simulink model "gtm_designFS"  (Simulink 8.0)
settings: Solver=ode3  SolverMode=SingleTasking  StartTime=0.0  StopTime=50  FixedStep=Timestep  MaxStep=0.1  MinStep=0.005  RelTol=1e-5
StopFcn:
  | MWSout=grabmws(bdroot);
  | MWSout.lastrun=datestr(now);
model workspace: external: MATLAB Code tmpfile_simWS.mat (data not in the file)
undefined symbols (not defined in the file): Aero, b, bias, INU_pos, LinearizeModeOn, runway_alt, sgn, sigbuilder_block, sldvsubsys, StatesInp, symmetric_aero_on, TrimModeOn
libraries: NoiseModel_lib x28, simulink x9, GTM_FS_aerolib x3, engine_GTM_FS_lib x2, Glenn_simp2_engine_lib x2, sensors_T2_lib x2, sldvlib x2, acparams_lib x1, auxvars_lib x1, eomlib x1, actuator_FS_lib x1, Coefficient_Evaluation_lib x1
(part 2 of 3)

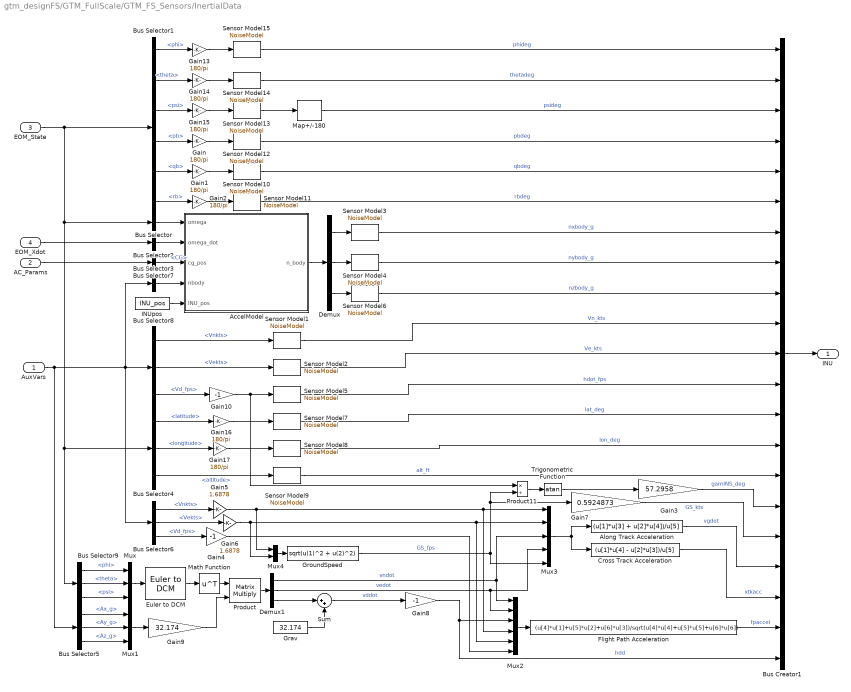
== system gtm_designFS/GTM_FullScale/GTM_FS_Sensors/InertialData ==
  AuxVars : Inport
  AC_Params : Inport  Port=2
  EOM_State : Inport  Port=3
  EOM_Xdot : Inport  Port=4
  AccelModel : MATLAB Function  TreatAsAtomicUnit=on
  Along Track Acceleration : Fcn  Expr=(u[1]*u[3] + u[2]*u[4])/u[5]
  Bus Creator1 : BusCreator  Inputs=21
  Bus Selector : BusSelector  OutputSignals=pb,qb,rb  OutputAsBus=on
  Bus Selector1 : BusSelector  OutputSignals=phi,theta,psi,pb,qb,rb
  Bus Selector2 : BusSelector  OutputSignals=pb_dot,qb_dot,rb_dot  OutputAsBus=on
  Bus Selector3 : BusSelector  OutputSignals=Ax_g,Ay_g,Az_g  OutputAsBus=on
  Bus Selector4 : BusSelector  OutputSignals=latitude,longitude,altitude
  Bus Selector5 : BusSelector  OutputSignals=Ax_g,Ay_g,Az_g
  Bus Selector6 : BusSelector  OutputSignals=Vnkts,Vekts,Vd_fps
  Bus Selector7 : BusSelector  OutputSignals=CG
  Bus Selector8 : BusSelector  OutputSignals=Vnkts,Vekts,Vd_fps
  Bus Selector9 : BusSelector  OutputSignals=phi,theta,psi
  Cross Track Acceleration : Fcn  Expr=(u[1]*u[4] - u[2]*u[3])/u[5]
  Demux : Demux  Outputs=3
  Demux1 : Demux  Outputs=3
  Euler to DCM : Euler_to_DCM_lib/Euler to DCM
  Flight Path Acceleration : Fcn  Expr=(u[4]*u[1]+u[5]*u[2]+u[6]*u[3])/sqrt(u[4]*u[4]+u[5]*u[5]+u[6]*u[6])
  Gain{,1..2,13..17} (8 alike) : Gain  Gain=180/pi
  Gain10 : Gain  Gain=-1
  Gain3 : Gain  Gain=57.2958  SaturateOnIntegerOverflow=on  OutDataTypeStr=Inherit: Same as input  ParamDataTypeStr=Inherit: Same as input
  Gain4 : Gain  Gain=-1
  Gain5 : Gain  Gain=1.6878
  Gain6 : Gain  Gain=1.6878
  Gain7 : Gain  Gain=0.5924873  SaturateOnIntegerOverflow=on  OutDataTypeStr=Inherit: Same as input  ParamDataTypeStr=Inherit: Same as input
  Gain8 : Gain  Gain=-1  SaturateOnIntegerOverflow=on  OutDataTypeStr=Inherit: Same as input  ParamDataTypeStr=Inherit: Same as input
  Gain9 : Gain  Gain=32.174  SaturateOnIntegerOverflow=on  OutDataTypeStr=Inherit: Same as input  ParamDataTypeStr=Inherit: Same as input
  Grav : Constant  Value=32.174  VectorParams1D=off
  GroundSpeed : Fcn  Expr=sqrt(u(1)^2 + u(2)^2)
  INUpos : Constant  Value=INU_pos  VectorParams1D=off
  Map+/-180 : sensors_T2_lib/GTM_T2/MIDG II 50 Hz/Map+//-180
  Math Function : Math  Operator=transpose  SaturateOnIntegerOverflow=on
  Mux : Mux  Inputs=3
  Mux1 : Mux  Inputs=3
  Mux2 : Mux  Inputs=6
  Mux3 : Mux  Inputs=5
  Mux4 : Mux  Inputs=2
  Product : Product  Multiplication=Matrix(*)  RndMeth=Zero
  Product11 : Product  Inputs=*/  SaturateOnIntegerOverflow=on  RndMeth=Zero  InputSameDT=on  OutDataTypeStr=Inherit: Same as first input
  Sensor Model1 : NoiseModel_lib/NoiseModel  noise_on=SensorNoise.On  sigma=SensorNoise.INU.Vn.Std  seed=878234  bias=SensorNoise.INU.Vn.Bias  scf=SensorNoise.INU.Vn.Scf
  Sensor Model10 : NoiseModel_lib/NoiseModel  noise_on=SensorNoise.On  sigma=SensorNoise.INU.qdeg.Std  seed=871234  bias=SensorNoise.INU.qdeg.Bias  scf=SensorNoise.INU.qdeg.Scf
  Sensor Model11 : NoiseModel_lib/NoiseModel  noise_on=SensorNoise.On  sigma=SensorNoise.INU.rdeg.Std  seed=878134  bias=SensorNoise.INU.rdeg.Bias  scf=SensorNoise.INU.rdeg.Scf
  Sensor Model12 : NoiseModel_lib/NoiseModel  noise_on=SensorNoise.On  sigma=SensorNoise.INU.pdeg.Std  seed=878233  bias=SensorNoise.INU.pdeg.Bias  scf=SensorNoise.INU.pdeg.Scf
  Sensor Model13 : NoiseModel_lib/NoiseModel  noise_on=SensorNoise.On  sigma=SensorNoise.INU.psi.Std  seed=878232  bias=SensorNoise.INU.psi.Bias  scf=SensorNoise.INU.psi.Scf
  Sensor Model14 : NoiseModel_lib/NoiseModel  noise_on=SensorNoise.On  sigma=SensorNoise.INU.theta.Std  seed=878231  bias=SensorNoise.INU.theta.Bias  scf=SensorNoise.INU.theta.Scf
  Sensor Model15 : NoiseModel_lib/NoiseModel  noise_on=SensorNoise.On  sigma=SensorNoise.INU.phi.Std  seed=878230  bias=SensorNoise.INU.phi.Bias  scf=SensorNoise.INU.phi.Scf
  Sensor Model2 : NoiseModel_lib/NoiseModel  noise_on=SensorNoise.On  sigma=SensorNoise.INU.Ve.Std  seed=8782345  bias=SensorNoise.INU.Ve.Bias  scf=SensorNoise.INU.Ve.Scf
  Sensor Model3 : NoiseModel_lib/NoiseModel  noise_on=SensorNoise.On  sigma=SensorNoise.INU.nxbody.Std  seed=878234  bias=SensorNoise.INU.nxbody.Bias  scf=SensorNoise.INU.nxbody.Scf
  Sensor Model4 : NoiseModel_lib/NoiseModel  noise_on=SensorNoise.On  sigma=SensorNoise.INU.nybody.Std  seed=8782345  bias=SensorNoise.INU.nybody.Bias  scf=SensorNoise.INU.nybody.Scf
  Sensor Model5 : NoiseModel_lib/NoiseModel  noise_on=SensorNoise.On  sigma=SensorNoise.INU.hdot.Std  seed=8782345  bias=SensorNoise.INU.hdot.Bias  scf=SensorNoise.INU.hdot.Scf
  Sensor Model6 : NoiseModel_lib/NoiseModel  noise_on=SensorNoise.On  sigma=SensorNoise.INU.nzbody.Std  seed=878236  bias=SensorNoise.INU.nzbody.Bias  scf=SensorNoise.INU.nzbody.Scf
  Sensor Model7 : NoiseModel_lib/NoiseModel  noise_on=SensorNoise.On  sigma=SensorNoise.INU.lat.Std  seed=8782345  bias=SensorNoise.INU.lat.Bias  scf=SensorNoise.INU.lat.Scf
  Sensor Model8 : NoiseModel_lib/NoiseModel  noise_on=SensorNoise.On  sigma=SensorNoise.INU.lon.Std  seed=8782345  bias=SensorNoise.INU.lon.Bias  scf=SensorNoise.INU.lon.Scf
  Sensor Model9 : NoiseModel_lib/NoiseModel  noise_on=SensorNoise.On  sigma=SensorNoise.INU.alt.Std  seed=8782345  bias=SensorNoise.INU.alt.Bias  scf=SensorNoise.INU.alt.Scf
  Sum : Sum  Inputs=|++
  Trigonometric Function : Trigonometry  Operator=atan
  INU : Outport
  wires:
  Bus Selector/1 -> AccelModel/1(omega)
  Bus Selector2/1 -> AccelModel/2(omega_dot)
  Bus Selector7/1 -> AccelModel/3(cg_pos)  "<CG>"
  Bus Selector3/1 -> AccelModel/4(nbody)
  AccelModel/1(n_body) -> Demux/1
  Demux/1 -> Sensor Model3/1
  Demux/2 -> Sensor Model4/1
  Demux/3 -> Sensor Model6/1
  Sensor Model1/1 -> Bus Creator1/10  "Vn_kts"
  Sensor Model2/1 -> Bus Creator1/11  "Ve_kts"
  Sensor Model9/1 -> Bus Creator1/15  "alt_ft"
  Sensor Model7/1 -> Bus Creator1/13  "lat_deg"
  Sensor Model8/1 -> Bus Creator1/14  "lon_deg"
  Bus Selector8/1 -> Sensor Model1/1  "<Vnkts>"
  Bus Selector8/2 -> Sensor Model2/1  "<Vekts>"
  Bus Selector8/3 -> Gain10/1  "<Vd_fps>"
  Bus Selector4/1 -> Gain16/1  "<latitude>"
  Bus Selector4/2 -> Gain17/1  "<longitude>"
  Bus Selector4/3 -> Sensor Model9/1  "<altitude>"
  Sensor Model5/1 -> Bus Creator1/12  "hdot_fps"
  Gain16/1 -> Sensor Model7/1
  Gain17/1 -> Sensor Model8/1
  EOM_Xdot/1 -> Bus Selector2/1
  AC_Params/1 -> Bus Selector7/1
  AuxVars/1 -> Bus Selector8/1, Bus Selector3/1, Bus Selector6/1, Bus Selector5/1
  EOM_State/1 -> Bus Selector1/1, Bus Selector/1, Bus Selector4/1, Bus Selector9/1
  Bus Selector1/1 -> Gain13/1  "<phi>"
  Bus Selector1/2 -> Gain14/1  "<theta>"
  Bus Selector1/3 -> Gain15/1  "<psi>"
  Bus Selector1/4 -> Gain/1  "<pb>"
  Bus Selector1/5 -> Gain1/1  "<qb>"
  Bus Selector1/6 -> Gain2/1  "<rb>"
  Gain2/1 -> Sensor Model11/1
  Gain1/1 -> Sensor Model10/1
  Gain/1 -> Sensor Model12/1
  Gain15/1 -> Sensor Model13/1
  Gain14/1 -> Sensor Model14/1
  Gain13/1 -> Sensor Model15/1
  Sensor Model13/1 -> Map+/-180/1
  Sensor Model15/1 -> Bus Creator1/1  "phideg"
  Sensor Model14/1 -> Bus Creator1/2  "thetadeg"
  Map+/-180/1 -> Bus Creator1/3  "psideg"
  Sensor Model12/1 -> Bus Creator1/4  "pbdeg"
  Sensor Model10/1 -> Bus Creator1/5  "qbdeg"
  Sensor Model11/1 -> Bus Creator1/6  "rbdeg"
  Sensor Model3/1 -> Bus Creator1/7  "nxbody_g"
  Sensor Model4/1 -> Bus Creator1/8  "nybody_g"
  Sensor Model6/1 -> Bus Creator1/9  "nzbody_g"
  INUpos/1 -> AccelModel/5(INU_pos)
  Mux/1 -> Euler to DCM/1
  Euler to DCM/1 -> Math Function/1
  Bus Selector5/1 -> Mux1/1  "<Ax_g>"
  Bus Selector5/2 -> Mux1/2  "<Ay_g>"
  Bus Selector5/3 -> Mux1/3  "<Az_g>"
  Math Function/1 -> Product/1
  Mux1/1 -> Gain9/1
  Mux3/1 -> Cross Track Acceleration/1, Along Track Acceleration/1
  Mux2/1 -> Flight Path Acceleration/1
  Trigonometric Function/1 -> Gain3/1
  Product11/1 -> Trigonometric Function/1
  Bus Selector6/3 -> Gain4/1  "<Vd_fps>"
  Bus Selector6/1 -> Gain5/1  "<Vnkts>"
  Bus Selector6/2 -> Gain6/1  "<Vekts>"
  Product/1 -> Demux1/1
  Bus Selector9/1 -> Mux/1  "<phi>"
  Bus Selector9/2 -> Mux/2  "<theta>"
  Bus Selector9/3 -> Mux/3  "<psi>"
  Gain5/1 -> Mux4/1, Mux3/1, Mux2/4
  Gain6/1 -> Mux4/2, Mux3/2, Mux2/5
  Mux4/1 -> GroundSpeed/1
  GroundSpeed/1 -> Mux3/5, Product11/2, Gain7/1  "GS_fps"
  Demux1/1 -> Mux3/3, Mux2/1  "vndot"
  Demux1/2 -> Mux3/4, Mux2/2  "vedot"
  Gain3/1 -> Bus Creator1/16  "gamINS_deg"
  Along Track Acceleration/1 -> Bus Creator1/18  "vgdot"
  Cross Track Acceleration/1 -> Bus Creator1/19  "xtkacc"
  Flight Path Acceleration/1 -> Bus Creator1/20  "fpaccel"
  Gain7/1 -> Bus Creator1/17  "GS_kts"
  Gain8/1 -> Mux2/3, Bus Creator1/21  "hdd"
  Gain4/1 -> Mux2/6
  Gain9/1 -> Product/2
  Demux1/3 -> Sum/1
  Grav/1 -> Sum/2
  Sum/1 -> Gain8/1  "vddot"
  Bus Creator1/1 -> INU/1
  Gain10/1 -> Sensor Model5/1, Product11/1

== system gtm_designFS/GTM_FullScale/GTM_FS_Sensors/SurfaceData ==
  SurfacePos : Inport
  Bus Creator : BusCreator  Inputs=22
  Bus Selector : BusSelector  OutputSignals=ELLOB,ELLIB,ELROB,ELRIB,AILL,AILR,RUDU,RUDL,FLAPLIB,FLAPLOB,FLAPRIB,FLAPROB  OutputAsBus=on
  Bus Selector1 : BusSelector  OutputSignals=ELLOB,ELLIB,ELROB,ELRIB,AILL,AILR,RUDU,RUDL,FLAPLIB,FLAPLOB,FLAPRIB,FLAPROB
  Bus Selector2 : BusSelector  OutputSignals=SPLLIB,SPLLOB,SPLRIB,SPLROB,STAB,GEAR,BRAKE,THROTL,THROTR,STEER
  Sensor Model5 : NoiseModel_lib/NoiseModel  noise_on=SensorNoise.On  sigma=SensorNoise.pots.Std  seed=878239  bias=SensorNoise.pots.Bias  scf=SensorNoise.pots.Scf
  Surface Labels : sensors_T2_lib/GTM_T2/Surface Pots/Surface Labels
  SurfPos : Outport
  wires:
  Bus Selector/1 -> Sensor Model5/1
  SurfacePos/1 -> Bus Selector/1, Bus Selector2/1
  Sensor Model5/1 -> Surface Labels/1
  Bus Selector1/1 -> Bus Creator/1  "<ELLOB>"
  Bus Selector1/2 -> Bus Creator/2  "<ELLIB>"
  Bus Selector1/3 -> Bus Creator/3  "<ELROB>"
  Bus Selector1/4 -> Bus Creator/4  "<ELRIB>"
  Bus Selector1/5 -> Bus Creator/5  "<AILL>"
  Bus Selector1/6 -> Bus Creator/6  "<AILR>"
  Bus Selector1/7 -> Bus Creator/7  "<RUDU>"
  Bus Selector1/8 -> Bus Creator/8  "<RUDL>"
  Bus Selector1/9 -> Bus Creator/9  "<FLAPLIB>"
  Bus Selector1/10 -> Bus Creator/10  "<FLAPLOB>"
  Bus Selector1/11 -> Bus Creator/11  "<FLAPRIB>"
  Bus Selector1/12 -> Bus Creator/12  "<FLAPROB>"
  Bus Selector2/1 -> Bus Creator/13  "<SPLLIB>"
  Bus Selector2/2 -> Bus Creator/14  "<SPLLOB>"
  Bus Selector2/3 -> Bus Creator/15  "<SPLRIB>"
  Bus Selector2/4 -> Bus Creator/16  "<SPLROB>"
  Bus Selector2/5 -> Bus Creator/17  "<STAB>"
  Bus Selector2/6 -> Bus Creator/18  "<GEAR>"
  Bus Selector2/7 -> Bus Creator/19  "<BRAKE>"
  Bus Selector2/8 -> Bus Creator/20  "<THROTL>"
  Bus Selector2/9 -> Bus Creator/21  "<THROTR>"
  Bus Selector2/10 -> Bus Creator/22  "<STEER>"
  Surface Labels/1 -> Bus Selector1/1
  Bus Creator/1 -> SurfPos/1

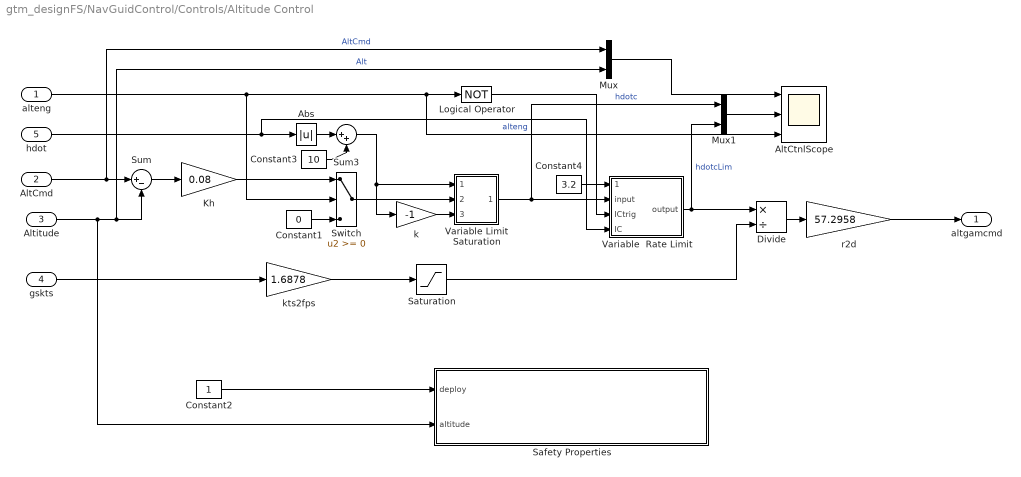
== system gtm_designFS/NavGuidControl/Controls/Altitude Control ==
  alteng : Inport
  AltCmd : Inport  Port=2
  Altitude : Inport  Port=3
  gskts : Inport  Port=4
  hdot : Inport  Port=5
  Abs : Abs  SaturateOnIntegerOverflow=on
  AltCtnlScope : Scope  NumInputPorts=3
      settings: TimeRange=30  YMin=10000~-5~0  YMax=10200~15~1  SaveName=ScopeData3
  Constant1 : Constant  Value=0
  Constant2 : Constant
  Constant3 : Constant  Value=10
  Constant4 : Constant  Value=3.2
  Divide : Product  Inputs=*/
  Kh : Gain  Gain=0.08
  Logical Operator : Logic  Operator=NOT
  Mux : Mux  Inputs=2
  Mux1 : Mux  Inputs=2
  Safety Properties : Subsystem  Tag=VerificationSubsystem  DisableCoverage=on  LoadFcn=sldvsubsys('check')  TreatAsAtomicUnit=on  SimViewingDevice=on  mask(VerificationSubsystem){}
      mask init:
      | sldvsubsys('maskInit');
      settings: CopyFcn=sldvsubsys('copy');  OpenFcn=open_system(gcb,'force');
      settings: PreSaveFcn=|
      | set_param(gcb,'SimViewingDevice','on');
      | sldvsubsys('check');
      mask Help: helpview(fullfile(docroot,'toolbox','sldv','sldv.map'),'verificationsubsystem')
      mask Display: image(imread('sldvicon_versubsys.png','BackGroundColor',[1 1 1]),'center');
  Saturation : Saturate  UpperLimit=1000  LowerLimit=0.0001
  Sum : Sum  Inputs=|+-
  Sum3 : Sum  Inputs=|++  SaturateOnIntegerOverflow=on  InputSameDT=on  OutDataTypeStr=Inherit: Same as first input
  Switch : Switch
  Variable  Rate Limit : Subsystem
  Variable Limit Saturation : Subsystem
  k : Gain  Gain=-1
  kts2fps : Gain  Gain=1.6878
  r2d : Gain  Gain=57.2958
  altgamcmd : Outport
  wires:
  Sum/1 -> Kh/1
  AltCmd/1 -> Sum/1, Mux/1  "AltCmd"
  Altitude/1 -> Safety Properties/2(altitude), Sum/2, Mux/2  "Alt"
  hdot/1 -> Abs/1, Variable  Rate Limit/4(IC)
  Abs/1 -> Sum3/1
  Constant3/1 -> Sum3/2
  k/1 -> Variable Limit Saturation/3(Lo_lim)
  Sum3/1 -> k/1, Variable Limit Saturation/1(up_lim)
  alteng/1 -> Switch/2, Logical Operator/1, AltCtnlScope/3  "alteng"
  gskts/1 -> kts2fps/1
  Divide/1 -> r2d/1
  r2d/1 -> altgamcmd/1
  Logical Operator/1 -> Variable  Rate Limit/3(ICtrig)
  Variable Limit Saturation/1(Out1) -> Variable  Rate Limit/2(input), Mux1/1  "hdotc"
  Constant4/1 -> Variable  Rate Limit/1(ratelim)
  Variable  Rate Limit/1(output) -> Divide/1, Mux1/2  "hdotcLim"
  kts2fps/1 -> Saturation/1
  Saturation/1 -> Divide/2
  Switch/1 -> Variable Limit Saturation/2(SigIn)
  Kh/1 -> Switch/1
  Constant1/1 -> Switch/3
  Mux/1 -> AltCtnlScope/1
  Mux1/1 -> AltCtnlScope/2
  Constant2/1 -> Safety Properties/1(deploy)

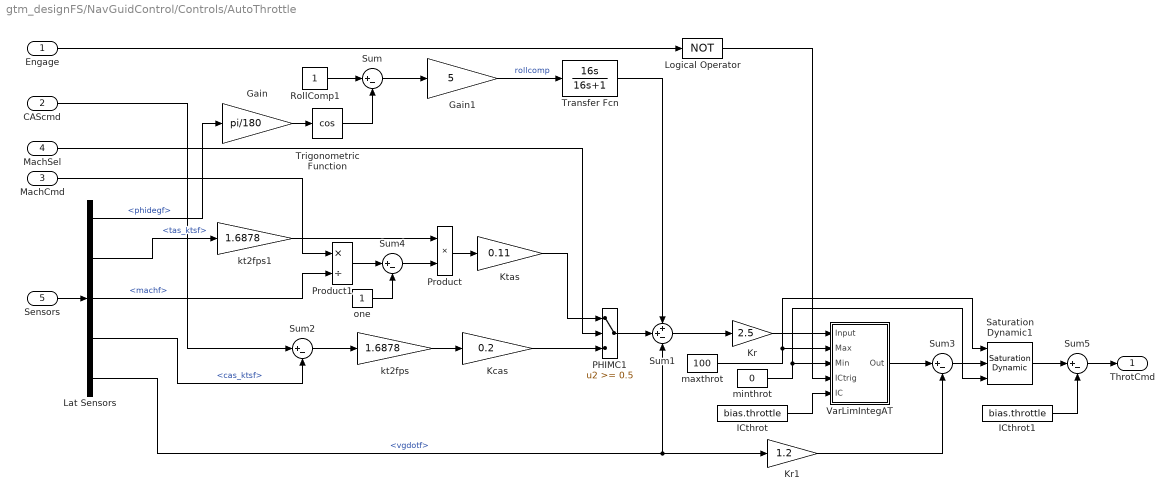
== system gtm_designFS/NavGuidControl/Controls/AutoThrottle ==
  Engage : Inport
  CAScmd : Inport  Port=2
  MachCmd : Inport  Port=3
  MachSel : Inport  Port=4
  Sensors : Inport  Port=5
  Gain : Gain  Gain=pi/180
  Gain1 : Gain  Gain=5
  ICthrot : Constant  Value=bias.throttle  SampleTime=-1
  ICthrot1 : Constant  Value=bias.throttle  SampleTime=-1
  Kcas : Gain  Gain=0.2
  Kr : Gain  Gain=2.5
  Kr1 : Gain  Gain=1.2
  Ktas : Gain  Gain=0.11
  Lat Sensors : BusSelector  OutputSignals=phidegf,tas_ktsf,machf,cas_ktsf,vgdotf
  Logical Operator : Logic  Operator=NOT  AllPortsSameDT=off  OutDataTypeStr=boolean
  PHIMC1 : Switch  Threshold=0.5  SampleTime=0.02  SaturateOnIntegerOverflow=on
  Product : Product  RndMeth=Zero
  Product1 : Product  Inputs=*/  RndMeth=Zero
  RollComp1 : Constant  SampleTime=-1
  Saturation Dynamic1 : simulink/Discontinuities/Saturation Dynamic  OutMin=[]  OutMax=[]  OutDataTypeStr=Inherit: Same as second input  OutDataType=sfix(16)  OutScaling=2^-10  DoSatur=off
  Sum{,2..5} (5 alike) : Sum  Inputs=|+-
  Sum1 : Sum  Inputs=++-
  Transfer Fcn : TransferFcn  Numerator=[16 0]  Denominator=[16 1]
  Trigonometric Function : Trigonometry  Operator=cos
  VarLimIntegAT : Subsystem
  kt2fps : Gain  Gain=1.6878
  kt2fps1 : Gain  Gain=1.6878
  maxthrot : Constant  Value=100  SampleTime=-1
  minthrot : Constant  Value=0  SampleTime=-1
  one : Constant  SampleTime=-1
  ThrotCmd : Outport
  wires:
  CAScmd/1 -> Sum2/1
  Sum2/1 -> kt2fps/1
  Sum1/1 -> Kr/1
  kt2fps/1 -> Kcas/1
  Kr/1 -> VarLimIntegAT/1(Input)
  Lat Sensors/5 -> Sum1/3, Kr1/1  "<vgdotf>"
  Kr1/1 -> Sum3/2
  Gain1/1 -> Transfer Fcn/1  "rollcomp"
  Sum/1 -> Gain1/1
  Trigonometric Function/1 -> Sum/2
  RollComp1/1 -> Sum/1
  Gain/1 -> Trigonometric Function/1
  Product1/1 -> Sum4/1
  one/1 -> Sum4/2
  Sum4/1 -> Product/2
  kt2fps1/1 -> Product/1
  Product/1 -> Ktas/1
  ICthrot/1 -> VarLimIntegAT/5(IC)
  Sum5/1 -> ThrotCmd/1
  ICthrot1/1 -> Sum5/2
  maxthrot/1 -> VarLimIntegAT/2(Max), Saturation Dynamic1/1
  minthrot/1 -> VarLimIntegAT/3(Min), Saturation Dynamic1/3
  VarLimIntegAT/1(Out) -> Sum3/1
  Sum3/1 -> Saturation Dynamic1/2
  Saturation Dynamic1/1 -> Sum5/1
  PHIMC1/1 -> Sum1/2
  Kcas/1 -> PHIMC1/3
  Ktas/1 -> PHIMC1/1
  Transfer Fcn/1 -> Sum1/1
  Sensors/1 -> Lat Sensors/1
  Lat Sensors/1 -> Gain/1  "<phidegf>"
  Lat Sensors/2 -> kt2fps1/1  "<tas_ktsf>"
  Lat Sensors/4 -> Sum2/2  "<cas_ktsf>"
  Logical Operator/1 -> VarLimIntegAT/4(ICtrig)
  Engage/1 -> Logical Operator/1
  MachSel/1 -> PHIMC1/2
  MachCmd/1 -> Product1/1
  Lat Sensors/3 -> Product1/2  "<machf>"

== system gtm_designFS/NavGuidControl/Controls/FPA Control ==
  engage : Inport
  gamcmd : Inport  Port=2
  gamma : Inport  Port=3
  thetadeg : Inport  Port=4
  VT : Inport  Port=5
  FPAScope : Scope  NumInputPorts=4
      settings: YMin=-1~-5~-2~-5  YMax=2~5~2~10  SaveName=ScopeData12
  Integ_FPA : Integrator  ExternalReset=level  InitialConditionSource=external  IgnoreLimit=on
  KIgamerr : Gain
  Kgamerr : Gain  Gain=1.4
  Logical Operator : Logic  Operator=NOT  AllPortsSameDT=off  OutDataTypeStr=boolean
  Mux : Mux  Inputs=2
  Mux1 : Mux  Inputs=2
  Product1 : Product  RndMeth=Zero
  Saturation Dynamic : simulink/Discontinuities/Saturation Dynamic  OutMin=[]  OutMax=[]  OutDataTypeStr=Inherit: Same as second input  OutDataType=fixdt(1, 16)  OutScaling=2^-10  DoSatur=off
  Sum : Sum  Inputs=|++
  Sum1 : Sum  Inputs=|+-
  Sum2 : Sum  Inputs=|+-
  hddLim : Constant  Value=4.83*57.2958
  kt2fps : Gain  Gain=1.6878
  m1 : Gain  Gain=-1
  PitchCmd : Outport
  wires:
  Sum1/1 -> PitchCmd/1, FPAScope/4  "PitchCmd"
  Kgamerr/1 -> Sum1/2, Sum/2
  Integ_FPA/1 -> Sum1/1
  gamma/1 -> Kgamerr/1, Sum2/2, Mux/2  "gamma"
  thetadeg/1 -> Sum/1
  Sum/1 -> Integ_FPA/3
  engage/1 -> Logical Operator/1, FPAScope/1  "engage"
  Logical Operator/1 -> Integ_FPA/2
  kt2fps/1 -> Product1/2
  hddLim/1 -> Product1/1
  Product1/1 -> Saturation Dynamic/1, m1/1
  VT/1 -> kt2fps/1
  Saturation Dynamic/1 -> Integ_FPA/1, Mux1/2  "gamerrlim"
  KIgamerr/1 -> Saturation Dynamic/2
  m1/1 -> Saturation Dynamic/3
  Sum2/1 -> KIgamerr/1, Mux1/1  "gamerr"
  gamcmd/1 -> Sum2/1, Mux/1  "gamcmd"
  Mux/1 -> FPAScope/2
  Mux1/1 -> FPAScope/3

== system gtm_designFS/NavGuidControl/Controls/FPAcmd ==
  Demux : Demux  Tag=STV Demux  Outputs=1
  FromWs : FromWorkspace  Tag=STV FromWs  VariableName=tuvar  SampleTime=0  SigBuilderData=DataTag0  VnvData=DataTag1
      SigBuilderData=|
      | common.afterFinalStr = 'Extrapolate'
      | common.sampleTime = 0
      | dataSet.timeRange = [0 10]
      | dataSet.name = 'Group 1'
      | sbobj.Groups.Name = 'Group 1'
      | sbobj.Groups.Signals.Name = 'Signal 1'
      | sbobj.Groups.Signals.XData = [0 1 1 6 10]
      | sbobj.Groups.Signals.YData = [0 0 1 1 1]
  Signal 1 : Outport  Tag=STV Outport
  wires:
  Demux/1 -> Signal 1/1
  FromWs/1 -> Demux/1

== system gtm_designFS/NavGuidControl/Controls/Heading Control ==
  HdgCmdMCP : Inport
  Heading : Inport  Port=2
  psidot : Inport  Port=3
  Vt : Inport  Port=4
  Roll : Inport  Port=5
  HdgCmdProcessor : Subsystem
  HdgRollCmdScope : Scope  NumInputPorts=8
      settings: YMin=-30~-30~-10~-10~-4~-10~0~-5  YMax=30~30~10~10~4~10~1~5  SaveName=ScopeData7
  Khdg : Gain  Gain=0.05
  Khdg1 : Gain
  Khdg2 : Gain
  Khdgrte : Gain  Gain=3
  Logical Operator : Logic  Operator=NOT  AllPortsSameDT=off  OutDataTypeStr=boolean
  MinMax : MinMax  Inputs=2
  MinMax1 : MinMax  Function=max  Inputs=2
  Mux : Mux  Inputs=2
  Sum : Sum  Inputs=|+-
  Sum1 : Sum  Inputs=|++
  Sum2 : Sum  Inputs=|+-
  Sum3 : Sum  Inputs=|--
  Sum4 : Sum  Inputs=+-|
  VarLimIntegIC : Subsystem
  sgn : Gain  Gain=-1
  RollCmd : Outport
  wires:
  Heading/1 -> Sum/2, HdgCmdProcessor/3(Heading)
  HdgCmdProcessor/1(HdgCmd) -> Sum/1, Mux/2  "psic"
  Sum/1 -> Khdg/1, HdgRollCmdScope/3  "psie"
  Khdg/1 -> Sum1/1
  Sum2/1 -> Sum1/2, HdgRollCmdScope/4  "psidote"
  HdgCmdProcessor/2(HdgRteCmd) -> Sum2/1, HdgRollCmdScope/2  "psidotc"
  psidot/1 -> Sum2/2
  Vt/1 -> HdgCmdProcessor/1(Vt)
  HdgCmdMCP/1 -> HdgCmdProcessor/2(HdgCmdMCP), Mux/1
  VarLimIntegIC/1(Out) -> RollCmd/1, Sum3/1, Sum4/2, HdgRollCmdScope/8  "phic"
  [rollLim] -> VarLimIntegIC/1(UpLim), sgn/1
  sgn/1 -> VarLimIntegIC/2(LoLim)
  [rollLim] -> Sum3/2, Sum4/1
  Sum1/1 -> Khdgrte/1
  MinMax1/1 -> MinMax/1, HdgRollCmdScope/6  "phidotcmx"
  MinMax/1 -> VarLimIntegIC/3(In), HdgRollCmdScope/7  "phidotcmn"
  [apeng] -> Logical Operator/1
  Sum3/1 -> Khdg1/1
  Sum4/1 -> Khdg2/1
  Khdg1/1 -> MinMax1/2
  Khdg2/1 -> MinMax/2
  Roll/1 -> VarLimIntegIC/5(IC)
  Khdgrte/1 -> MinMax1/1, HdgRollCmdScope/5  "phidotc"
  Logical Operator/1 -> VarLimIntegIC/4(Trig)
  Mux/1 -> HdgRollCmdScope/1

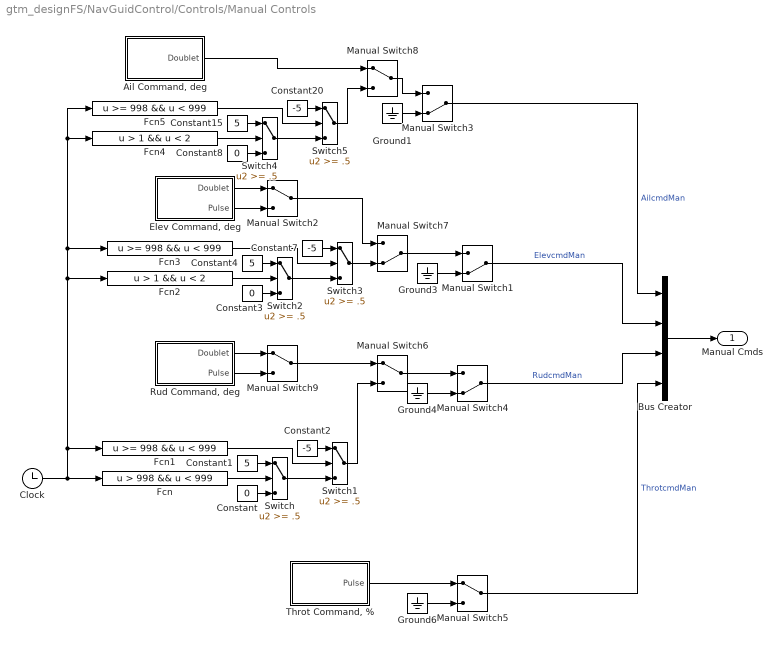
== system gtm_designFS/NavGuidControl/Controls/Manual Controls ==
  "Ail Command, deg" : Subsystem  Tag=STV Subsys  LoadFcn=sigbuilder_block('load');  StartFcn=sigbuilder_block('start');  StopFcn=sigbuilder_block('stop');  ClipboardFcn=sigbuilder_block('clipboard');  mask(Sigbuilder block){}
      mask help: Sigbuilder GUI
      mask init:
      | if ~strcmp(get_param(bdroot(gcbh),'SimulationStatus'),'stopped') tuvar = sigbuilder_block('maskInit'); end
      settings: CopyFcn=sigbuilder_block('copy');  DeleteFcn=sigbuilder_block('delete');  ModelCloseFcn=sigbuilder_block('modelClose');  PreSaveFcn=sigbuilder_block('preSave');  PauseFcn=sigbuilder_block('pause')  ContinueFcn=sigbuilder_block('continue')  NameChangeFcn=sigbuilder_block('namechange');  OpenFcn=sigbuilder_block('open',[20.16 261.12 550.08 400.32 ]);  CloseFcn=sigbuilder_block('close');
      mask Display: plot(0,0,100,100,[10,10,40,40,10],[80,20,20,80,80],[40,10],[50,50], [40,27,10],[65,72,56],[40,25,25,10],[28,28,43,43]);
  Bus Creator : BusCreator
  Clock : Clock
  Constant : Constant  Value=0
  Constant1 : Constant  Value=5
  Constant15 : Constant  Value=5
  Constant2 : Constant  Value=-5
  Constant20 : Constant  Value=-5
  Constant3 : Constant  Value=0
  Constant4 : Constant  Value=5
  Constant7 : Constant  Value=-5
  Constant8 : Constant  Value=0
  "Elev Command, deg" : Subsystem  Tag=STV Subsys  LoadFcn=sigbuilder_block('load');  StartFcn=sigbuilder_block('start');  StopFcn=sigbuilder_block('stop');  ClipboardFcn=sigbuilder_block('clipboard');  mask(Sigbuilder block){}
      mask help: Sigbuilder GUI
      mask init:
      | if ~strcmp(get_param(bdroot(gcbh),'SimulationStatus'),'stopped') tuvar = sigbuilder_block('maskInit'); end
      settings: CopyFcn=sigbuilder_block('copy');  DeleteFcn=sigbuilder_block('delete');  ModelCloseFcn=sigbuilder_block('modelClose');  PreSaveFcn=sigbuilder_block('preSave');  PauseFcn=sigbuilder_block('pause')  ContinueFcn=sigbuilder_block('continue')  NameChangeFcn=sigbuilder_block('namechange');  OpenFcn=sigbuilder_block('open',[550.08 198.72 550.08 400.32 ]);  CloseFcn=sigbuilder_block('close');
      mask Display: plot(0,0,100,100,[10,10,40,40,10],[80,20,20,80,80],[40,10],[50,50], [40,27,10],[65,72,56],[40,25,25,10],[28,28,43,43]);
  Fcn : Fcn  Expr=u > 998 && u < 999
  Fcn1 : Fcn  Expr=u >= 998 && u < 999
  Fcn2 : Fcn  Expr=u > 1 && u < 2
  Fcn3 : Fcn  Expr=u >= 998 && u < 999
  Fcn4 : Fcn  Expr=u > 1 && u < 2
  Fcn5 : Fcn  Expr=u >= 998 && u < 999
  Ground{1,3..4,6} (4 alike) : Ground
  Manual Switch{1,3..4,7} (4 alike) : ManualSwitch  CurrentSetting=0
  Manual Switch{2,5..6,8..9} (5 alike) : ManualSwitch
  "Rud Command, deg" : Subsystem  Tag=STV Subsys  LoadFcn=sigbuilder_block('load');  StartFcn=sigbuilder_block('start');  StopFcn=sigbuilder_block('stop');  ClipboardFcn=sigbuilder_block('clipboard');  mask(Sigbuilder block){}
      mask help: Sigbuilder GUI
      mask init:
      | if ~strcmp(get_param(bdroot(gcbh),'SimulationStatus'),'stopped') tuvar = sigbuilder_block('maskInit'); end
      settings: CopyFcn=sigbuilder_block('copy');  DeleteFcn=sigbuilder_block('delete');  ModelCloseFcn=sigbuilder_block('modelClose');  PreSaveFcn=sigbuilder_block('preSave');  PauseFcn=sigbuilder_block('pause')  ContinueFcn=sigbuilder_block('continue')  NameChangeFcn=sigbuilder_block('namechange');  OpenFcn=sigbuilder_block('open',[437.6 199.2 550.4 400 ]);  CloseFcn=sigbuilder_block('close');
      mask Display: plot(0,0,100,100,[10,10,40,40,10],[80,20,20,80,80],[40,10],[50,50], [40,27,10],[65,72,56],[40,25,25,10],[28,28,43,43]);
  Switch{,1..5} (6 alike) : Switch  Threshold=.5
  "Throt Command, %" : Subsystem  Tag=STV Subsys  LoadFcn=sigbuilder_block('load');  StartFcn=sigbuilder_block('start');  StopFcn=sigbuilder_block('stop');  ClipboardFcn=sigbuilder_block('clipboard');  mask(Sigbuilder block){}
      mask help: Sigbuilder GUI
      mask init:
      | if ~strcmp(get_param(bdroot(gcbh),'SimulationStatus'),'stopped') tuvar = sigbuilder_block('maskInit'); end
      settings: CopyFcn=sigbuilder_block('copy');  DeleteFcn=sigbuilder_block('delete');  ModelCloseFcn=sigbuilder_block('modelClose');  PreSaveFcn=sigbuilder_block('preSave');  PauseFcn=sigbuilder_block('pause')  ContinueFcn=sigbuilder_block('continue')  NameChangeFcn=sigbuilder_block('namechange');  OpenFcn=sigbuilder_block('open',[436.656 201.841 549.567 399.685 ]);  CloseFcn=sigbuilder_block('close');
      mask Display: plot(0,0,100,100,[10,10,40,40,10],[80,20,20,80,80],[40,10],[50,50], [40,27,10],[65,72,56],[40,25,25,10],[28,28,43,43]);
  Manual Cmds : Outport
  wires:
  Ground1/1 -> Manual Switch3/2
  Ground3/1 -> Manual Switch1/2
  "Elev Command, deg"/1(Doublet) -> Manual Switch2/1
  "Elev Command, deg"/2(Pulse) -> Manual Switch2/2
  Ground4/1 -> Manual Switch4/2
  Ground6/1 -> Manual Switch5/2
  "Throt Command, %"/1(Pulse) -> Manual Switch5/1
  Fcn/1 -> Switch/2
  Constant1/1 -> Switch/1
  Constant/1 -> Switch/3
  Switch/1 -> Switch1/3
  Constant2/1 -> Switch1/1
  Fcn1/1 -> Switch1/2
  Clock/1 -> Fcn/1, Fcn1/1, Fcn2/1, Fcn3/1, Fcn5/1, Fcn4/1
  Manual Switch6/1 -> Manual Switch4/1
  Switch1/1 -> Manual Switch6/2
  Fcn2/1 -> Switch2/2
  Constant4/1 -> Switch2/1
  Constant3/1 -> Switch2/3
  Switch2/1 -> Switch3/3
  Constant7/1 -> Switch3/1
  Fcn3/1 -> Switch3/2
  Manual Switch7/1 -> Manual Switch1/1
  Switch3/1 -> Manual Switch7/2
  Manual Switch2/1 -> Manual Switch7/1
  Fcn4/1 -> Switch4/2
  Constant15/1 -> Switch4/1
  Constant8/1 -> Switch4/3
  Switch4/1 -> Switch5/3
  Constant20/1 -> Switch5/1
  Fcn5/1 -> Switch5/2
  Manual Switch8/1 -> Manual Switch3/1
  Switch5/1 -> Manual Switch8/2
  "Ail Command, deg"/1(Doublet) -> Manual Switch8/1
  Manual Switch3/1 -> Bus Creator/1  "AilcmdMan"
  Manual Switch1/1 -> Bus Creator/2  "ElevcmdMan"
  Manual Switch4/1 -> Bus Creator/3  "RudcmdMan"
  Manual Switch5/1 -> Bus Creator/4  "ThrotcmdMan"
  Bus Creator/1 -> Manual Cmds/1
  "Rud Command, deg"/1(Doublet) -> Manual Switch9/1
  "Rud Command, deg"/2(Pulse) -> Manual Switch9/2
  Manual Switch9/1 -> Manual Switch6/1

== system gtm_designFS/NavGuidControl/Controls/ManualPitchcmd ==
  Thetafiltdeg : Inport
  Constant : Constant  Value=3
  Constant1 : Constant  Value=0
  Integrator +/- 50 deg/sec : Integrator  InitialConditionSource=external  LimitOutput=on  UpperSaturationLimit=50  LowerSaturationLimit=-50
  ManualPitchScope : Scope  NumInputPorts=6
      settings: YMin=-5~-5~-5~-5~-5~-5  YMax=5~5~5~5~5~5  SaveName=ScopeData8
  Multiport Switch : MultiPortSwitch
  PS Gain deg/sec : Gain  Gain=50
  "PS Shaping " : Fcn  Expr=u(1)*abs(u(1))^1.0
  PS deadband +/- 0.01 : DeadZone  LowerValue=-0.01  UpperValue=0.01  SaturateOnIntegerOverflow=on
  PS limits +/- 1 : Saturate  UpperLimit=1  LowerLimit=-1
  Pitchcmd : Subsystem  Tag=STV Subsys  LoadFcn=sigbuilder_block('load');  StartFcn=sigbuilder_block('start');  StopFcn=sigbuilder_block('stop');  ClipboardFcn=sigbuilder_block('clipboard');  mask(Sigbuilder block){}
      mask help: Sigbuilder GUI
      mask init:
      | if ~strcmp(get_param(bdroot(gcbh),'SimulationStatus'),'stopped') tuvar = sigbuilder_block('maskInit'); end
      settings: CopyFcn=sigbuilder_block('copy');  DeleteFcn=sigbuilder_block('delete');  ModelCloseFcn=sigbuilder_block('modelClose');  PreSaveFcn=sigbuilder_block('preSave');  PauseFcn=sigbuilder_block('pause')  ContinueFcn=sigbuilder_block('continue')  NameChangeFcn=sigbuilder_block('namechange');  OpenFcn=sigbuilder_block('open',[159.36 418.56 676.8 484.8 ]);  CloseFcn=sigbuilder_block('close');
      mask Display: plot(0,0,100,100,[10,10,40,40,10],[80,20,20,80,80],[40,10],[50,50], [40,27,10],[65,72,56],[40,25,25,10],[28,28,43,43]);
  PitchCmd : Outport
  wires:
  Pitchcmd/2(Signal 2) -> Multiport Switch/4
  Pitchcmd/1(Signal 1) -> Multiport Switch/3
  Constant1/1 -> Multiport Switch/2
  Constant/1 -> Multiport Switch/1
  Multiport Switch/1 -> ManualPitchScope/1, PS limits +/- 1/1  "stick"
  Thetafiltdeg/1 -> Integrator +/- 50 deg/sec/2
  Integrator +/- 50 deg/sec/1 -> ManualPitchScope/6, PitchCmd/1  "pitchcmd"
  PS Gain deg/sec/1 -> ManualPitchScope/5, Integrator +/- 50 deg/sec/1  "q_cmd"
  PS deadband +/- 0.01/1 -> ManualPitchScope/3, "PS Shaping "/1  "stkdb"
  PS limits +/- 1/1 -> ManualPitchScope/2, PS deadband +/- 0.01/1  "stklim"
  "PS Shaping "/1 -> ManualPitchScope/4, PS Gain deg/sec/1  "stkshape"

== system gtm_designFS/NavGuidControl/Controls/ManualRollcmd ==
  rollfiltdeg : Inport
  Constant1 : Constant  Value=0
  Integrator +/- 225 deg/sec : Integrator  InitialConditionSource=external  LimitOutput=on  UpperSaturationLimit=225  LowerSaturationLimit=-225
  ManualRollScope : Scope  NumInputPorts=6
      settings: YMin=-5~-5~-5~-5~-5~-5  YMax=5~5~5~5~5~5  SaveName=ScopeData9
  Multiport Switch : MultiPortSwitch
  RS Gain deg/sec : Gain  Gain=225
  "RS Shaping " : Fcn  Expr=u(1)*abs(u(1))^1.0
  RS deadband +/- 0.01 : DeadZone  LowerValue=-0.01  UpperValue=0.01  SaturateOnIntegerOverflow=on
  RS limits +/- 1 : Saturate  UpperLimit=1  LowerLimit=-1
  Rollcmd : Subsystem  Tag=STV Subsys  LoadFcn=sigbuilder_block('load');  StartFcn=sigbuilder_block('start');  StopFcn=sigbuilder_block('stop');  ClipboardFcn=sigbuilder_block('clipboard');  mask(Sigbuilder block){}
      mask help: Sigbuilder GUI
      mask init:
      | if ~strcmp(get_param(bdroot(gcbh),'SimulationStatus'),'stopped') tuvar = sigbuilder_block('maskInit'); end
      settings: CopyFcn=sigbuilder_block('copy');  DeleteFcn=sigbuilder_block('delete');  ModelCloseFcn=sigbuilder_block('modelClose');  PreSaveFcn=sigbuilder_block('preSave');  PauseFcn=sigbuilder_block('pause')  ContinueFcn=sigbuilder_block('continue')  NameChangeFcn=sigbuilder_block('namechange');  OpenFcn=sigbuilder_block('open',[159.36 418.56 676.8 484.8 ]);  CloseFcn=sigbuilder_block('close');
      mask Display: plot(0,0,100,100,[10,10,40,40,10],[80,20,20,80,80],[40,10],[50,50], [40,27,10],[65,72,56],[40,25,25,10],[28,28,43,43]);
  portselect : Constant
  RollCmd : Outport
  wires:
  rollfiltdeg/1 -> Integrator +/- 225 deg/sec/2
  Rollcmd/2(Signal 2) -> Multiport Switch/4
  Rollcmd/1(Signal 1) -> Multiport Switch/3
  Constant1/1 -> Multiport Switch/2
  Multiport Switch/1 -> ManualRollScope/1, RS limits +/- 1/1  "rollstick"
  Integrator +/- 225 deg/sec/1 -> ManualRollScope/6, RollCmd/1  "rollcmd"
  RS Gain deg/sec/1 -> ManualRollScope/5, Integrator +/- 225 deg/sec/1  "p_cmd"
  RS deadband +/- 0.01/1 -> ManualRollScope/3, "RS Shaping "/1  "rstkdb"
  RS limits +/- 1/1 -> ManualRollScope/2, RS deadband +/- 0.01/1  "rstklim"
  "RS Shaping "/1 -> ManualRollScope/4, RS Gain deg/sec/1  "rstkshape"
  portselect/1 -> Multiport Switch/1

== system gtm_designFS/NavGuidControl/Controls/Pitch InnerLoop ==
  PitchCmd : Inport
  Pitch : Inport  Port=2
  qdeg : Inport  Port=3
  CAS : Inport  Port=4
  Kcas : Lookup  InputValues=[0 120 350 500]  Table=[1.0 1.0 0.3 0.3]
  Kpitch : Gain  Gain=2
  Kwo : Gain  Gain=0.5
  Mux : Mux  Inputs=2
  PitchScope : Scope  NumInputPorts=6
      settings: YMin=-2~-2~-2~-20~-20~0  YMax=10~2~2~20~20~1.2  SaveName=ScopeData11
  Product : Product  RndMeth=Zero
  Sum : Sum  Inputs=|+-
  Sum1 : Sum  Inputs=|-+
  Transfer Fcn : TransferFcn  Numerator=[16 0]  Denominator=[16 1]
  ElevCmd : Outport
  wires:
  Sum/1 -> Kpitch/1, PitchScope/2  "Pitcherror"
  Pitch/1 -> Sum/2, Mux/2
  Kpitch/1 -> Sum1/1
  qdeg/1 -> Transfer Fcn/1
  Transfer Fcn/1 -> Kwo/1
  CAS/1 -> Kcas/1
  Sum1/1 -> Product/1, PitchScope/4  "dec"
  Kcas/1 -> Product/2, PitchScope/6  "Kcas"
  Product/1 -> ElevCmd/1, PitchScope/5  "elevcmd"
  Kwo/1 -> Sum1/2, PitchScope/3  "qdegwo"
  PitchCmd/1 -> Sum/1, Mux/1  "Pitchcmd"
  Mux/1 -> PitchScope/1

== system gtm_designFS/NavGuidControl/Controls/PitchCmd ==
  Pitchcmd1 : Subsystem  Tag=STV Subsys  LoadFcn=sigbuilder_block('load');  StartFcn=sigbuilder_block('start');  StopFcn=sigbuilder_block('stop');  ClipboardFcn=sigbuilder_block('clipboard');  mask(Sigbuilder block){}
      mask help: Sigbuilder GUI
      mask init:
      | if ~strcmp(get_param(bdroot(gcbh),'SimulationStatus'),'stopped') tuvar = sigbuilder_block('maskInit'); end
      settings: CopyFcn=sigbuilder_block('copy');  DeleteFcn=sigbuilder_block('delete');  ModelCloseFcn=sigbuilder_block('modelClose');  PreSaveFcn=sigbuilder_block('preSave');  PauseFcn=sigbuilder_block('pause')  ContinueFcn=sigbuilder_block('continue')  NameChangeFcn=sigbuilder_block('namechange');  OpenFcn=sigbuilder_block('open',[437.6 199.2 550.4 400 ]);  CloseFcn=sigbuilder_block('close');
      mask Display: plot(0,0,100,100,[10,10,40,40,10],[80,20,20,80,80],[40,10],[50,50], [40,27,10],[65,72,56],[40,25,25,10],[28,28,43,43]);
  Sum1 : Sum  Inputs=|++
  Trim Pitch : Constant  Value=StatesInp(11)*180/pi
  Cmd : Outport
  wires:
  Pitchcmd1/1(Signal 1) -> Sum1/1
  Trim Pitch/1 -> Sum1/2
  Sum1/1 -> Cmd/1

== system gtm_designFS/NavGuidControl/Controls/Roll InnerLoop ==
  note: orig =[0 60 140]
  note: orig = 0.25
  note: orig = 0.8
  RollCmd : Inport
  Roll : Inport  Port=2
  pdeg : Inport  Port=3
  CAS : Inport  Port=4
  Kcas : Lookup  InputValues=[0 120 350 500]  Table=[1.0 1.0 0.3 0.3]
  Kphierr : Gain  Gain=0.5
  Product : Product  RndMeth=Zero
  Roll_IL_scope : Scope  NumInputPorts=7
      settings: YMin=-30~-30~-10~-10~-4~-10~0  YMax=30~30~10~10~4~10~1  SaveName=ScopeData5
  Sum : Sum  Inputs=|+-
  Sum1 : Sum  Inputs=|+-
  rollrate_IL : ZeroPole  Zeros=0  Poles=-0.5  Gain=0.00645
  AilCmd : Outport
  wires:
  Product/1 -> AilCmd/1, Roll_IL_scope/6  "ailcmd"
  Kcas/1 -> Product/2, Roll_IL_scope/7  "kcas"
  Sum1/1 -> Product/1
  CAS/1 -> Kcas/1
  rollrate_IL/1 -> Sum1/2, Roll_IL_scope/5  "pdegwo"
  pdeg/1 -> rollrate_IL/1, Roll_IL_scope/4  "pdeg"
  Kphierr/1 -> Sum1/1
  Roll/1 -> Sum/2, Roll_IL_scope/2  "roll"
  Sum/1 -> Kphierr/1, Roll_IL_scope/3  "rollerr"
  RollCmd/1 -> Sum/1, Roll_IL_scope/1  "rollcmd"

== system gtm_designFS/NavGuidControl/Controls/Signal Builder ==
  Demux : Demux  Tag=STV Demux  Outputs=3
  FromWs : FromWorkspace  Tag=STV FromWs  VariableName=tuvar  SampleTime=0  SigBuilderData=DataTag16  VnvData=DataTag17
      SigBuilderData=|
      | common.afterFinalStr = 'Extrapolate'
      | common.sampleTime = 0
      | dataSet.timeRange = [0 60]
      | dataSet.name = 'Group 1'
      | sbobj.Groups.Name = 'Group 1'
      | sbobj.Groups.Signals(1).Name = 'Signal 1'
      | sbobj.Groups.Signals(1).XData = [0 1 1 60]
      | sbobj.Groups.Signals(1).YData = [0 0 30 30]
      | sbobj.Groups.Signals(2).Name = 'Signal 2'
      | sbobj.Groups.Signals(2).XData = [0 1 1 60]
      | sbobj.Groups.Signals(2).YData = [0 0 50 50]
      | sbobj.Groups.Signals(3).Name = 'Signal 3'
      | sbobj.Groups.Signals(3).XData = [0 1 1 60]
      | sbobj.Groups.Signals(3).YData = [0 0 90 90]
  Signal 1 : Outport  Tag=STV Outport
  Signal 2 : Outport  Tag=STV Outport  Port=2
  Signal 3 : Outport  Tag=STV Outport  Port=3
  wires:
  Demux/1 -> Signal 1/1
  FromWs/1 -> Demux/1
  Demux/2 -> Signal 2/1
  Demux/3 -> Signal 3/1

== system gtm_designFS/NavGuidControl/Controls/Stall Protect ==
  In1 : Inport
  Out1 : Outport
  wires:
  In1/1 -> Out1/1

== system gtm_designFS/NavGuidControl/Controls/Yaw Damper ==
  rdeg : Inport
  CAS : Inport  Port=2
  Kcas : Lookup  InputValues=[0 120 350 500]  Table=[1.0 1.0 0.3 0.3]
  Kr : Gain  Gain=1.25
  Product : Product  RndMeth=Zero
  YD_wo : TransferFcn  Numerator=[1 0]  Denominator=[1 10]
  RudCmd : Outport
  wires:
  rdeg/1 -> Kr/1
  CAS/1 -> Kcas/1
  Kcas/1 -> Product/2
  Product/1 -> RudCmd/1
  Kr/1 -> YD_wo/1
  YD_wo/1 -> Product/1

== system gtm_designFS/NavGuidControl/SignalProcessing/EULER_RATES ==
  Sensors : Inport
  Bus Creator : BusCreator  Inputs=3
  Bus Creator1 : BusCreator
  Bus Selector23 : BusSelector  OutputSignals=pbdegf,qbdegf,rdegf,phidegf,thetadegf
  Product{,1..2,4..5} (5 alike) : Product  SaturateOnIntegerOverflow=on  OutDataTypeStr=Inherit: Same as first input
  Product3 : Product  Inputs=*/  SaturateOnIntegerOverflow=on  OutDataTypeStr=Inherit: Same as first input
  Product6 : Product  Inputs=*/  SaturateOnIntegerOverflow=on  OutDataTypeStr=Inherit: Same as first input
  Sum : Sum  Inputs=|++  SaturateOnIntegerOverflow=on
  Sum1 : Sum  Inputs=|++  SaturateOnIntegerOverflow=on
  Sum2 : Sum  Inputs=|+-  SaturateOnIntegerOverflow=on
  Trigonometric Function1 : Trigonometry  Operator=cos
  Trigonometric Function2 : Trigonometry
  Trigonometric Function3 : Trigonometry
  Trigonometric Function4 : Trigonometry  Operator=cos
  d2r : Gain  Gain=pi/180
  d2r1 : Gain  Gain=pi/180
  Rates : Outport
  SC_phithet : Outport  Port=2
  wires:
  Bus Creator1/1 -> SC_phithet/1  "SCphithet"
  d2r1/1 -> Trigonometric Function3/1, Trigonometric Function4/1
  d2r/1 -> Trigonometric Function2/1, Trigonometric Function1/1
  Sensors/1 -> Bus Selector23/1
  Bus Selector23/4 -> d2r/1  "<phidegf>"
  Bus Selector23/5 -> d2r1/1  "<thetadegf>"
  Bus Selector23/2 -> Product/1, Product4/1  "<qbdegf>"
  Trigonometric Function2/1 -> Bus Creator1/1, Product5/2, Product/2  "sphi"
  Product/1 -> Sum/1
  Bus Selector23/3 -> Product1/1, Product5/1  "<rdegf>"
  Trigonometric Function1/1 -> Bus Creator1/2, Product4/2, Product1/2  "cphi"
  Product1/1 -> Sum/2
  Bus Selector23/1 -> Sum1/1  "<pbdegf>"
  Trigonometric Function3/1 -> Bus Creator1/3, Product3/1  "stheta"
  Trigonometric Function4/1 -> Bus Creator1/4, Product6/2, Product3/2  "ctheta"
  Sum/1 -> Product2/1, Product6/1
  Product3/1 -> Product2/2
  Product2/1 -> Sum1/2
  Sum1/1 -> Bus Creator/1  "phidotdeg"
  Bus Creator/1 -> Rates/1  "EulerRates"
  Product4/1 -> Sum2/1
  Product5/1 -> Sum2/2
  Sum2/1 -> Bus Creator/2  "thetdotdeg"
  Product6/1 -> Bus Creator/3  "psidotdeg"

== system gtm_designFS/NavGuidControl/SignalProcessing/LP_Filter1 ==
  In : Inport
  Gain : Gain  Gain=6*pi
  Integrator : Integrator  InitialConditionSource=external
  Sum : Sum  Inputs=|+-
  Out : Outport
  wires:
  Integrator/1 -> Out/1, Sum/2
  Gain/1 -> Integrator/1
  In/1 -> Sum/1, Integrator/2
  Sum/1 -> Gain/1

== system gtm_designFS/NavGuidControl/SignalProcessing/LP_Filter10 ==
  In : Inport
  Gain : Gain  Gain=6*pi
  Integrator : Integrator  InitialConditionSource=external
  Sum : Sum  Inputs=|+-
  Out : Outport
  wires:
  Integrator/1 -> Out/1, Sum/2
  Gain/1 -> Integrator/1
  In/1 -> Sum/1, Integrator/2
  Sum/1 -> Gain/1

== system gtm_designFS/NavGuidControl/SignalProcessing/LP_Filter11 ==
  In : Inport
  Gain : Gain  Gain=6*pi
  Integrator : Integrator  InitialConditionSource=external
  Sum : Sum  Inputs=|+-
  Out : Outport
  wires:
  Sum/1 -> Gain/1
  In/1 -> Integrator/2, Sum/1
  Gain/1 -> Integrator/1
  Integrator/1 -> Sum/2, Out/1

== system gtm_designFS/NavGuidControl/SignalProcessing/LP_Filter12 ==
  In : Inport
  Gain : Gain  Gain=6*pi
  Integrator : Integrator  InitialConditionSource=external
  Sum : Sum  Inputs=|+-
  Out : Outport
  wires:
  Integrator/1 -> Out/1, Sum/2
  Gain/1 -> Integrator/1
  In/1 -> Sum/1, Integrator/2
  Sum/1 -> Gain/1

== system gtm_designFS/NavGuidControl/SignalProcessing/LP_Filter13 ==
  In : Inport
  Gain : Gain  Gain=6*pi
  Integrator : Integrator  InitialConditionSource=external
  Sum : Sum  Inputs=|+-
  Out : Outport
  wires:
  Sum/1 -> Gain/1
  In/1 -> Integrator/2, Sum/1
  Gain/1 -> Integrator/1
  Integrator/1 -> Sum/2, Out/1

== system gtm_designFS/NavGuidControl/SignalProcessing/LP_Filter14 ==
  In : Inport
  Gain : Gain  Gain=6*pi
  Integrator : Integrator  InitialConditionSource=external
  Sum : Sum  Inputs=|+-
  Out : Outport
  wires:
  Integrator/1 -> Out/1, Sum/2
  Gain/1 -> Integrator/1
  In/1 -> Sum/1, Integrator/2
  Sum/1 -> Gain/1

== system gtm_designFS/NavGuidControl/SignalProcessing/LP_Filter15 ==
  In : Inport
  Gain : Gain  Gain=6*pi
  Integrator : Integrator  InitialConditionSource=external
  Sum : Sum  Inputs=|+-
  Out : Outport
  wires:
  Sum/1 -> Gain/1
  In/1 -> Integrator/2, Sum/1
  Gain/1 -> Integrator/1
  Integrator/1 -> Sum/2, Out/1

== system gtm_designFS/NavGuidControl/SignalProcessing/LP_Filter16 ==
  In : Inport
  Gain : Gain  Gain=6*pi
  Integrator : Integrator  InitialConditionSource=external
  Sum : Sum  Inputs=|+-
  Out : Outport
  wires:
  Integrator/1 -> Out/1, Sum/2
  Gain/1 -> Integrator/1
  In/1 -> Sum/1, Integrator/2
  Sum/1 -> Gain/1

== system gtm_designFS/NavGuidControl/SignalProcessing/LP_Filter17 ==
  In : Inport
  Gain : Gain  Gain=6*pi
  Integrator : Integrator  InitialConditionSource=external
  Sum : Sum  Inputs=|+-
  Out : Outport
  wires:
  Sum/1 -> Gain/1
  In/1 -> Integrator/2, Sum/1
  Gain/1 -> Integrator/1
  Integrator/1 -> Sum/2, Out/1

== system gtm_designFS/NavGuidControl/SignalProcessing/LP_Filter18 ==
  In : Inport
  Gain : Gain  Gain=6*pi
  Integrator : Integrator
  Sum : Sum  Inputs=|+-
  Out : Outport
  wires:
  Integrator/1 -> Out/1, Sum/2
  Gain/1 -> Integrator/1
  In/1 -> Sum/1
  Sum/1 -> Gain/1

== system gtm_designFS/NavGuidControl/SignalProcessing/LP_Filter19 ==
  In : Inport
  Gain : Gain  Gain=6*pi
  Integrator : Integrator
  Sum : Sum  Inputs=|+-
  Out : Outport
  wires:
  Sum/1 -> Gain/1
  In/1 -> Sum/1
  Gain/1 -> Integrator/1
  Integrator/1 -> Sum/2, Out/1

== system gtm_designFS/NavGuidControl/SignalProcessing/LP_Filter2 ==
  In : Inport
  Gain : Gain  Gain=6*pi
  Integrator : Integrator  InitialConditionSource=external
  Sum : Sum  Inputs=|+-
  Out : Outport
  wires:
  Sum/1 -> Gain/1
  In/1 -> Integrator/2, Sum/1
  Gain/1 -> Integrator/1
  Integrator/1 -> Sum/2, Out/1

== system gtm_designFS/NavGuidControl/SignalProcessing/LP_Filter20 ==
  In : Inport
  Gain : Gain  Gain=6*pi
  Integrator : Integrator
  Sum : Sum  Inputs=|+-
  Out : Outport
  wires:
  Integrator/1 -> Out/1, Sum/2
  Gain/1 -> Integrator/1
  In/1 -> Sum/1
  Sum/1 -> Gain/1

== system gtm_designFS/NavGuidControl/SignalProcessing/LP_Filter21 ==
  In : Inport
  Gain : Gain  Gain=6*pi
  Integrator : Integrator
  Sum : Sum  Inputs=|+-
  Out : Outport
  wires:
  Sum/1 -> Gain/1
  In/1 -> Sum/1
  Gain/1 -> Integrator/1
  Integrator/1 -> Sum/2, Out/1

== system gtm_designFS/NavGuidControl/SignalProcessing/LP_Filter22 ==
  In : Inport
  Gain : Gain  Gain=6*pi
  Integrator : Integrator  InitialConditionSource=external
  Sum : Sum  Inputs=|+-
  Out : Outport
  wires:
  Integrator/1 -> Out/1, Sum/2
  Gain/1 -> Integrator/1
  In/1 -> Sum/1, Integrator/2
  Sum/1 -> Gain/1

== system gtm_designFS/NavGuidControl/SignalProcessing/LP_Filter23 ==
  In : Inport
  Gain : Gain  Gain=6*pi
  Integrator : Integrator  InitialConditionSource=external
  Sum : Sum  Inputs=|+-
  Out : Outport
  wires:
  Sum/1 -> Gain/1
  In/1 -> Integrator/2, Sum/1
  Gain/1 -> Integrator/1
  Integrator/1 -> Sum/2, Out/1

== system gtm_designFS/NavGuidControl/SignalProcessing/LP_Filter24 ==
  In : Inport
  Gain : Gain  Gain=6*pi
  Integrator : Integrator  InitialConditionSource=external
  Sum : Sum  Inputs=|+-
  Out : Outport
  wires:
  Integrator/1 -> Out/1, Sum/2
  Gain/1 -> Integrator/1
  In/1 -> Sum/1, Integrator/2
  Sum/1 -> Gain/1

== system gtm_designFS/NavGuidControl/SignalProcessing/LP_Filter25 ==
  In : Inport
  Gain : Gain  Gain=6*pi
  Integrator : Integrator  InitialConditionSource=external
  Sum : Sum  Inputs=|+-
  Out : Outport
  wires:
  Sum/1 -> Gain/1
  In/1 -> Integrator/2, Sum/1
  Gain/1 -> Integrator/1
  Integrator/1 -> Sum/2, Out/1

== system gtm_designFS/NavGuidControl/SignalProcessing/LP_Filter26 ==
  In : Inport
  Gain : Gain  Gain=6*pi
  Integrator : Integrator  InitialConditionSource=external
  Sum : Sum  Inputs=|+-
  Out : Outport
  wires:
  Integrator/1 -> Out/1, Sum/2
  Gain/1 -> Integrator/1
  In/1 -> Sum/1, Integrator/2
  Sum/1 -> Gain/1

== system gtm_designFS/NavGuidControl/SignalProcessing/LP_Filter27 ==
  In : Inport
  Gain : Gain  Gain=6*pi
  Integrator : Integrator  InitialConditionSource=external
  Sum : Sum  Inputs=|+-
  Out : Outport
  wires:
  Sum/1 -> Gain/1
  In/1 -> Integrator/2, Sum/1
  Gain/1 -> Integrator/1
  Integrator/1 -> Sum/2, Out/1

== system gtm_designFS/NavGuidControl/SignalProcessing/LP_Filter28 ==
  In : Inport
  Gain : Gain  Gain=6*pi
  Integrator : Integrator  InitialConditionSource=external
  Sum : Sum  Inputs=|+-
  Out : Outport
  wires:
  Integrator/1 -> Out/1, Sum/2
  Gain/1 -> Integrator/1
  In/1 -> Sum/1, Integrator/2
  Sum/1 -> Gain/1

== system gtm_designFS/NavGuidControl/SignalProcessing/LP_Filter3 ==
  In : Inport
  Gain : Gain  Gain=6*pi
  Integrator : Integrator  InitialConditionSource=external
  Sum : Sum  Inputs=|+-
  Out : Outport
  wires:
  Sum/1 -> Gain/1
  In/1 -> Integrator/2, Sum/1
  Gain/1 -> Integrator/1
  Integrator/1 -> Sum/2, Out/1

== system gtm_designFS/NavGuidControl/SignalProcessing/LP_Filter4 ==
  In : Inport
  Gain : Gain  Gain=6*pi
  Integrator : Integrator  InitialConditionSource=external
  Sum : Sum  Inputs=|+-
  Out : Outport
  wires:
  Integrator/1 -> Out/1, Sum/2
  Gain/1 -> Integrator/1
  In/1 -> Sum/1, Integrator/2
  Sum/1 -> Gain/1

== system gtm_designFS/NavGuidControl/SignalProcessing/LP_Filter5 ==
  In : Inport
  Gain : Gain  Gain=6*pi
  Integrator : Integrator  InitialConditionSource=external
  Sum : Sum  Inputs=|+-
  Out : Outport
  wires:
  Sum/1 -> Gain/1
  In/1 -> Integrator/2, Sum/1
  Gain/1 -> Integrator/1
  Integrator/1 -> Sum/2, Out/1

== system gtm_designFS/NavGuidControl/SignalProcessing/LP_Filter6 ==
  In : Inport
  Gain : Gain  Gain=6*pi
  Integrator : Integrator  InitialConditionSource=external
  Sum : Sum  Inputs=|+-
  Out : Outport
  wires:
  Integrator/1 -> Out/1, Sum/2
  Gain/1 -> Integrator/1
  In/1 -> Sum/1, Integrator/2
  Sum/1 -> Gain/1

== system gtm_designFS/NavGuidControl/SignalProcessing/LP_Filter7 ==
  In : Inport
  Gain : Gain  Gain=6*pi
  Integrator : Integrator
  Sum : Sum  Inputs=|+-
  Out : Outport
  wires:
  Sum/1 -> Gain/1
  In/1 -> Sum/1
  Gain/1 -> Integrator/1
  Integrator/1 -> Sum/2, Out/1

== system gtm_designFS/NavGuidControl/SignalProcessing/LP_Filter8 ==
  In : Inport
  Gain : Gain  Gain=6*pi
  Integrator : Integrator
  Sum : Sum  Inputs=|+-
  Out : Outport
  wires:
  Integrator/1 -> Out/1, Sum/2
  Gain/1 -> Integrator/1
  In/1 -> Sum/1
  Sum/1 -> Gain/1

== system gtm_designFS/NavGuidControl/SignalProcessing/LP_Filter9 ==
  In : Inport
  Gain : Gain  Gain=6*pi
  Integrator : Integrator  InitialConditionSource=external
  Sum : Sum  Inputs=|+-
  Out : Outport
  wires:
  Sum/1 -> Gain/1
  In/1 -> Integrator/2, Sum/1
  Gain/1 -> Integrator/1
  Integrator/1 -> Sum/2, Out/1

== system gtm_designFS/NavGuidControl/Controls/Altitude Control/Safety Properties ==
  note: If altitude>100000 feets, deploy cannot be true.
  deploy : Inport
  altitude : Inport  Port=2
  Compare To Constant : simulink/Logic and Bit Operations/Compare To Constant  relop=>  const=100000  OutDataTypeStr=uint8  ZeroCross=off
  Implies : sldvlib/Verification Utilities/Implies
  altitude valid : Assertion  Enabled=on
  wires:
  Implies/1 -> altitude valid/1
  Compare To Constant/1 -> Implies/1
  deploy/1 -> Implies/2
  altitude/1 -> Compare To Constant/1

== system gtm_designFS/NavGuidControl/Controls/Altitude Control/Variable  Rate Limit ==
  ratelim : Inport
  input : Inport  Port=2
  ICtrig : Inport  Port=3
  IC : Inport  Port=4
  Gain : Gain  Gain=20  SaturateOnIntegerOverflow=on  OutDataTypeStr=Inherit: Same as input  ParamDataTypeStr=Inherit: Same as input
  Gain1 : Gain  Gain=-1  SaturateOnIntegerOverflow=on  OutDataTypeStr=Inherit: Same as input  ParamDataTypeStr=Inherit: Same as input
  Integrator : Integrator  ExternalReset=level  InitialConditionSource=external  IgnoreLimit=on
  Sum2 : Sum  Inputs=|+-  SaturateOnIntegerOverflow=on
  Variable Limit Saturation : Subsystem
  output : Outport
  wires:
  Sum2/1 -> Gain/1
  Gain/1 -> Variable Limit Saturation/2(SigIn)
  ratelim/1 -> Gain1/1, Variable Limit Saturation/1(up_lim)
  Gain1/1 -> Variable Limit Saturation/3(Lo_lim)
  Variable Limit Saturation/1(Out1) -> Integrator/1
  Integrator/1 -> Sum2/2, output/1
  input/1 -> Sum2/1
  ICtrig/1 -> Integrator/2
  IC/1 -> Integrator/3

== system gtm_designFS/NavGuidControl/Controls/Altitude Control/Variable Limit Saturation ==
  up_lim : Inport
  SigIn : Inport  Port=2
  Lo_lim : Inport  Port=3
  Enforce low lim : MinMax  Function=max  Inputs=2
  Enforce up lim : MinMax  Inputs=2
  Out1 : Outport
  wires:
  Lo_lim/1 -> Enforce low lim/1
  SigIn/1 -> Enforce low lim/2
  Enforce low lim/1 -> Enforce up lim/1
  up_lim/1 -> Enforce up lim/2
  Enforce up lim/1 -> Out1/1

== system gtm_designFS/NavGuidControl/Controls/AutoThrottle/VarLimIntegAT ==
  Input : Inport
  Max : Inport  Port=2
  Min : Inport  Port=3
  ICtrig : Inport  Port=4
  IC : Inport  Port=5
  Constant1 : Constant  Value=0  SampleTime=-1
  Constant2 : Constant  Value=0  SampleTime=-1
  Constant3 : Constant  Value=0  SampleTime=-1
  Integrator1 : Integrator  ExternalReset=level  InitialConditionSource=external
  Logical Operator1 : Logic  Operator=OR
  Logical Operator2 : Logic
  Logical Operator3 : Logic
  Relational Operator1 : RelationalOperator  Operator=<=  InputSameDT=on
  Relational Operator2 : RelationalOperator  InputSameDT=on
  Relational Operator3 : RelationalOperator  Operator=>  InputSameDT=on
  Relational Operator4 : RelationalOperator  Operator=<  InputSameDT=on
  Switch1 : Switch  Threshold=0.1  SaturateOnIntegerOverflow=on  InputSameDT=on
  Out : Outport
  wires:
  IC/1 -> Integrator1/3
  ICtrig/1 -> Integrator1/2
  Min/1 -> Relational Operator1/2
  Max/1 -> Relational Operator2/2
  Constant3/1 -> Relational Operator4/2
  Input/1 -> Switch1/3, Relational Operator3/1, Relational Operator4/1
  Logical Operator3/1 -> Logical Operator1/2
  Relational Operator4/1 -> Logical Operator3/2
  Relational Operator1/1 -> Logical Operator3/1
  Constant2/1 -> Relational Operator3/2
  Logical Operator2/1 -> Logical Operator1/1
  Relational Operator3/1 -> Logical Operator2/2
  Relational Operator2/1 -> Logical Operator2/1
  Logical Operator1/1 -> Switch1/2
  Integrator1/1 -> Relational Operator2/1, Relational Operator1/1, Out/1
  Switch1/1 -> Integrator1/1
  Constant1/1 -> Switch1/1
